simulink model "SimulBoucle"  (R2024b)
settings: Solver=ode45  StartTime=0.0  StopTime=1000  RelTol=1e-7  EnableMultiTasking=on
values from neighbouring files (symbols this model uses):
  Controleur = tf(gc_num, gc_den)    [auto_identification.m]
  procede = tf(gp_num, gp_den, 'InputDelay', gp_retard)    [auto_identification.m]
settings Model: Creator=LiberT  LastModifiedBy=Mathieu Bouchard
settings SolverCC: AlgebraicLoopSolver=TrustRegion
settings DataIOCC: LimitDataPoints=on  SaveFormat=Array  SignalLoggingSaveFormat=ModelDataLogs  ReturnWorkspaceOutputs=off
settings OptimizationCC: BlockReduction=off  BooleanDataType=off  ExpressionDepthLimit=2147483647  InitFltsAndDblsToZero=on  LifeSpan=inf
settings DebuggingCC: SaveWithParameterizedLinksMsg=none  UnderspecifiedInitializationDetection=Classic  MergeDetectMultiDrivingBlocksExec=none  SignalResolutionControl=TryResolveAllWithWarning  MultiTaskDSMMsg=warning  MultiTaskCondExecSysMsg=none  FcnCallInpInsideContextMsg=warning  UnconnectedInputMsg=warning  UnconnectedOutputMsg=warning  UnconnectedLineMsg=warning  StateNameClashWarn=warning  SFUnexpectedBacktrackingDiag=warning  SFNoUnconditionalDefaultTransitionDiag=warning  SFExecutionAtInitializationDiag=none  ArithmeticOperatorsInVariantConditions=warning
settings HardwareCC: ProdBitPerPointer=32  ProdBitPerSizeT=32  ProdBitPerPtrDiffT=32  ProdLargestAtomicFloat=None  ProdIntDivRoundTo=Undefined  ProdEndianess=Unspecified  ProdWordSize=32  ProdHWDeviceType=32-bit Generic  TargetUnknown=on
settings ModelReferenceCC: EnableRefExpFcnMdlSchedulingChecks=on  PropagateSignalLabelsOutOfModel=off
settings SFSimCC: SimUseLocalCustomCode=off  CustomCodeUndefinedFunction=UseInterfaceOnly
settings RTWCC: RTWUseLocalCustomCode=off  GPUComputeCapability=3.5
settings CodeAppCC: StateflowObjectComments=on
settings GRTTargetCC: TargetFcnLib=ansi_tfl_tmw.mat  TargetLangStandard=C89/C90 (ANSI)  ModelReferenceCompliant=off  CompOptLevelCompliant=off  CombineOutputUpdateFcns=off  MatFileLogging=off  GRTInterface=on
settings ConfigComp: CovMetricSettings=dw  CovSaveCumulativeToWorkspaceVar=on  CovSaveSingleToWorkspaceVar=on  CovExternalEMLEnable=off

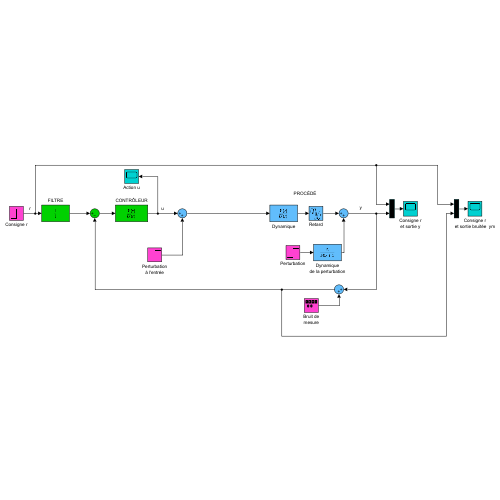
[thumbnail: Simulink's stored preview of the top-level diagram]
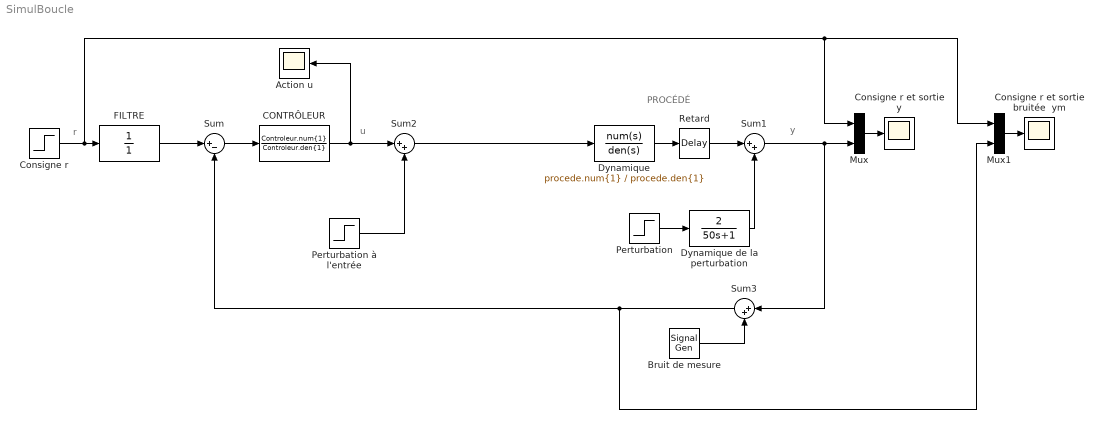
== system SimulBoucle ==
  note: PROCÉDÉ
  note: r
  note: u
  note: y
  Action u : Scope
  Bruit de mesure : SignalGenerator  Amplitude=0  Units=rad/sec
  CONTRÔLEUR : TransferFcn  Numerator=Controleur.num{1}  Denominator=Controleur.den{1}
  Consigne r : Step  Time=10  SampleTime=0
  Consigne r et sortie bruitée  ym : Scope
  Consigne r et sortie y : Scope
  Dynamique : TransferFcn  Numerator=procede.num{1}  Denominator=procede.den{1}
  Dynamique de la perturbation : TransferFcn  Numerator=2  Denominator=[50 1]
  FILTRE : TransferFcn  Numerator=1  Denominator=1
  Mux : Mux  Inputs=2
  Mux1 : Mux  Inputs=2
  Perturbation : Step  Time=300  After=0  SampleTime=0
  Perturbation à l'entrée : Step  Time=30  After=0  SampleTime=0
  Retard : TransportDelay  DelayTime=procede.InputDelay  BufferSize=10000
  Sum : Sum  Inputs=|+-  InputSameDT=on  SaturateOnIntegerOverflow=on  OutDataTypeStr=Inherit: Same as first input
  Sum1 : Sum  Inputs=|++  InputSameDT=on  SaturateOnIntegerOverflow=on  OutDataTypeStr=Inherit: Same as first input
  Sum2 : Sum  Inputs=|++  InputSameDT=on  SaturateOnIntegerOverflow=on  OutDataTypeStr=Inherit: Same as first input
  Sum3 : Sum  Inputs=|++  InputSameDT=on  SaturateOnIntegerOverflow=on  OutDataTypeStr=Inherit: Same as first input
  wires:
  Sum/1 -> CONTRÔLEUR/1
  CONTRÔLEUR/1 -> Action u/1, Sum2/1
  Sum1/1 -> Mux/2, Sum3/1
  Mux/1 -> Consigne r et sortie y/1
  Dynamique/1 -> Retard/1
  Retard/1 -> Sum1/1
  Sum2/1 -> Dynamique/1
  Perturbation à l'entrée/1 -> Sum2/2
  FILTRE/1 -> Sum/1
  Consigne r/1 -> FILTRE/1, Mux/1, Mux1/1
  Sum3/1 -> Mux1/2, Sum/2
  Bruit de mesure/1 -> Sum3/2
  Perturbation/1 -> Dynamique de la perturbation/1
  Dynamique de la perturbation/1 -> Sum1/2
  Mux1/1 -> Consigne r et sortie bruitée  ym/1
